simulink library "motor_interface_lib"  (R2022b)
settings: Solver=VariableStepAuto  StartTime=0.0  StopTime=10.0  RelTol=1e-3
undefined symbols (not defined in the file): MI_STATUSES
settings Model: Creator=dr_pa  LastModifiedBy=LinF

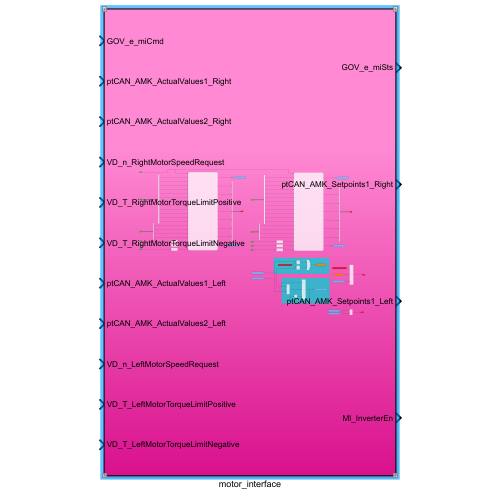
[thumbnail: Simulink's stored preview of the top-level diagram]
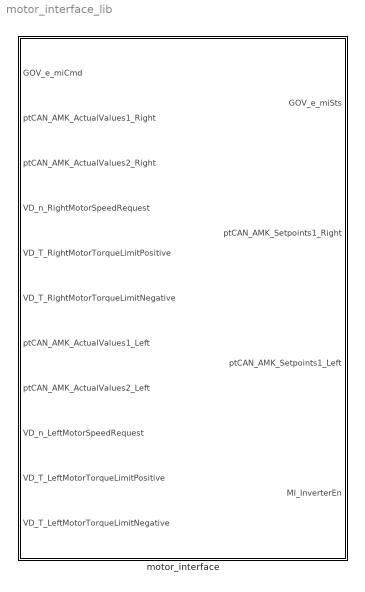
== system motor_interface_lib ==
  motor_interface : Subsystem

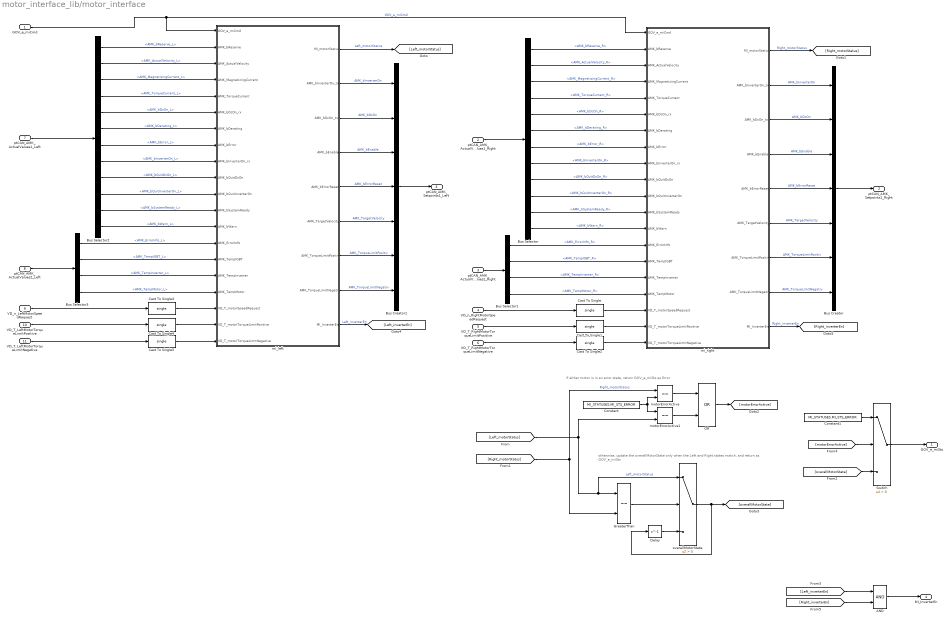
== system motor_interface_lib/motor_interface ==
  note: otherwise, update the overallMotorState only when the Left and Right states match, and return as GOV_e_miSts
  note: if either motor is in an error state, return GOV_e_miSts as Error
  GOV_e_miCmd : Inport
  ptCAN_AMK_ActualValues1_Right : Inport  Port=2
  ptCAN_AMK_ActualValues2_Right : Inport  Port=3
  VD_n_RightMotorSpeedRequest : Inport  Port=4
  VD_T_RightMotorTorqueLimitPositive : Inport  Port=5
  VD_T_RightMotorTorqueLimitNegative : Inport  Port=6
  ptCAN_AMK_ActualValues1_Left : Inport  Port=7
  ptCAN_AMK_ActualValues2_Left : Inport  Port=8
  VD_n_LeftMotorSpeedRequest : Inport  Port=9
  VD_T_LeftMotorTorqueLimitPositive : Inport  Port=10
  VD_T_LeftMotorTorqueLimitNegative : Inport  Port=11
  AND : Logic  AllPortsSameDT=off  OutDataTypeStr=boolean
  Bus Creator : BusCreator  Inputs=7
  Bus Creator1 : BusCreator  Inputs=7
  Bus Selector : BusSelector  OutputSignals=AMK_bReserve_R,AMK_ActualVelocity_R,AMK_MagnetizingCurrent_R,AMK_TorqueCurrent_R,AMK_bDcOn_R,AMK_bDerating_R,AMK_bError_R,AMK_bInverterOn_R,AMK_bQuitDcOn_R,AMK_bQuitInverterOn_R,AMK_bSystemReady_R,AMK_bWarn_R
  Bus Selector1 : BusSelector  OutputSignals=AMK_ErrorInfo_R,AMK_TempIGBT_R,AMK_TempInverter_R,AMK_TempMotor_R
  Bus Selector2 : BusSelector  OutputSignals=AMK_bReserve_L,AMK_ActualVelocity_L,AMK_MagnetizingCurrent_L,AMK_TorqueCurrent_L,AMK_bDcOn_L,AMK_bDerating_L,AMK_bError_L,AMK_bInverterOn_L,AMK_bQuitDcOn_L,AMK_bQuitInverterOn_L,AMK_bSystemReady_L,AMK_bWarn_L
  Bus Selector3 : BusSelector  OutputSignals=AMK_ErrorInfo_L,AMK_TempIGBT_L,AMK_TempInverter_L,AMK_TempMotor_L
  Cast To Single{,1..5} (6 alike) : DataTypeConversion  OutDataTypeStr=single  SaturateOnIntegerOverflow=off  RndMeth=Floor
  Constant : Constant  Value=MI_STATUSES.MI_STS_ERROR  OutDataTypeStr=Enum: MI_STATUSES
  Constant1 : Constant  Value=MI_STATUSES.MI_STS_ERROR  OutDataTypeStr=Enum: MI_STATUSES
  Delay : Delay  DelayLength=1  InitialCondition=MI_STATUSES.OFF
  GreaterThan : RelationalOperator  Operator===  OutDataTypeStr=boolean  RndMeth=Simplest  InputSameDT=off
  OR : Logic  Operator=OR  IconShape=distinctive  AllPortsSameDT=off  OutDataTypeStr=boolean
  Switch : Switch  Criteria=u2 > Threshold  SaturateOnIntegerOverflow=off  InputSameDT=off
  mi_left : Stateflow chart  TreatAsAtomicUnit=on
  mi_right : Stateflow chart  TreatAsAtomicUnit=on
  motorErrorActive : RelationalOperator  Operator===  OutDataTypeStr=boolean  RndMeth=Simplest  InputSameDT=off
  motorErrorActive1 : RelationalOperator  Operator===  OutDataTypeStr=boolean  RndMeth=Simplest  InputSameDT=off
  overallMotorState : Switch  Criteria=u2 > Threshold  SaturateOnIntegerOverflow=off  InputSameDT=off
  GOV_e_miSts : Outport
  ptCAN_AMK_Setpoints1_Right : Outport  Port=2
  ptCAN_AMK_Setpoints1_Left : Outport  Port=3
  MI_InverterEn : Outport  Port=4
  wires:
  [Right_inverterEn] -> AND/2
  [Left_inverterEn] -> AND/1
  mi_right/9(MI_InverterEn) -> [Right_inverterEn]  "Right_inverterEn"
  mi_left/9(MI_InverterEn) -> [Left_inverterEn]  "Left_inverterEn"
  AND/1 -> MI_InverterEn/1
  Bus Selector3/4 -> mi_left/17(AMK_TempMotor)  "<AMK_TempMotor_L>"
  Bus Selector3/3 -> mi_left/16(AMK_TempInverter)  "<AMK_TempInverter_L>"
  Bus Selector3/2 -> mi_left/15(AMK_TempIGBT)  "<AMK_TempIGBT_L>"
  Bus Selector3/1 -> mi_left/14(AMK_ErrorInfo)  "<AMK_ErrorInfo_L>"
  Bus Selector2/12 -> mi_left/13(AMK_bWarn)  "<AMK_bWarn_L>"
  Bus Selector2/11 -> mi_left/12(AMK_bSystemReady)  "<AMK_bSystemReady_L>"
  Bus Selector2/10 -> mi_left/11(AMK_bQuitInverterOn)  "<AMK_bQuitInverterOn_L>"
  Bus Selector2/9 -> mi_left/10(AMK_bQuitDcOn)  "<AMK_bQuitDcOn_L>"
  Bus Selector2/8 -> mi_left/9(AMK_bInverterOn_rx)  "<AMK_bInverterOn_L>"
  Bus Selector2/7 -> mi_left/8(AMK_bError)  "<AMK_bError_L>"
  Bus Selector2/6 -> mi_left/7(AMK_bDerating)  "<AMK_bDerating_L>"
  Bus Selector2/5 -> mi_left/6(AMK_bDcOn_rx)  "<AMK_bDcOn_L>"
  Bus Selector2/4 -> mi_left/5(AMK_TorqueCurrent)  "<AMK_TorqueCurrent_L>"
  Bus Selector2/3 -> mi_left/4(AMK_MagnetizingCurrent)  "<AMK_MagnetizingCurrent_L>"
  Bus Selector2/2 -> mi_left/3(AMK_ActualVelocity)  "<AMK_ActualVelocity_L>"
  Cast To Single5/1 -> mi_left/20(VD_T_motorTorqueLimitNegative)
  Cast To Single4/1 -> mi_left/19(VD_T_motorTorqueLimitPositive)
  Cast To Single3/1 -> mi_left/18(VD_T_motorSpeedRequest)
  Cast To Single2/1 -> mi_right/20(VD_T_motorTorqueLimitNegative)
  Cast To Single1/1 -> mi_right/19(VD_T_motorTorqueLimitPositive)
  Cast To Single/1 -> mi_right/18(VD_T_motorSpeedRequest)
  GOV_e_miCmd/1 -> mi_left/1(GOV_e_miCmd), mi_right/1(GOV_e_miCmd)  "GOV_e_miCmd"
  ptCAN_AMK_ActualValues1_Right/1 -> Bus Selector/1
  Bus Selector/2 -> mi_right/3(AMK_ActualVelocity)  "<AMK_ActualVelocity_R>"
  Bus Selector/3 -> mi_right/4(AMK_MagnetizingCurrent)  "<AMK_MagnetizingCurrent_R>"
  Bus Selector/4 -> mi_right/5(AMK_TorqueCurrent)  "<AMK_TorqueCurrent_R>"
  Bus Selector/5 -> mi_right/6(AMK_bDcOn_rx)  "<AMK_bDcOn_R>"
  Bus Selector/6 -> mi_right/7(AMK_bDerating)  "<AMK_bDerating_R>"
  Bus Selector/7 -> mi_right/8(AMK_bError)  "<AMK_bError_R>"
  Bus Selector/8 -> mi_right/9(AMK_bInverterOn_rx)  "<AMK_bInverterOn_R>"
  Bus Selector/9 -> mi_right/10(AMK_bQuitDcOn)  "<AMK_bQuitDcOn_R>"
  Bus Selector/10 -> mi_right/11(AMK_bQuitInverterOn)  "<AMK_bQuitInverterOn_R>"
  Bus Selector/11 -> mi_right/12(AMK_bSystemReady)  "<AMK_bSystemReady_R>"
  Bus Selector/12 -> mi_right/13(AMK_bWarn)  "<AMK_bWarn_R>"
  Bus Selector/1 -> mi_right/2(AMK_bReserve)  "<AMK_bReserve_R>"
  ptCAN_AMK_ActualValues2_Right/1 -> Bus Selector1/1
  Bus Selector1/1 -> mi_right/14(AMK_ErrorInfo)  "<AMK_ErrorInfo_R>"
  Bus Selector1/2 -> mi_right/15(AMK_TempIGBT)  "<AMK_TempIGBT_R>"
  Bus Selector1/3 -> mi_right/16(AMK_TempInverter)  "<AMK_TempInverter_R>"
  Bus Selector1/4 -> mi_right/17(AMK_TempMotor)  "<AMK_TempMotor_R>"
  Bus Creator/1 -> ptCAN_AMK_Setpoints1_Right/1
  mi_right/2(AMK_bInverterOn_tx) -> Bus Creator/1  "AMK_bInverterOn"
  mi_right/4(AMK_bEnable) -> Bus Creator/3  "AMK_bEnable"
  mi_right/6(AMK_TargetVelocity) -> Bus Creator/5  "AMK_TargetVelocity"
  mi_right/3(AMK_bDcOn_tx) -> Bus Creator/2  "AMK_bDcOn"
  mi_right/5(AMK_bErrorReset) -> Bus Creator/4  "AMK_bErrorReset"
  mi_left/1(MI_motorStatus) -> [Left_motorStatus]  "Left_motorStatus"
  mi_right/1(MI_motorStatus) -> [Right_motorStatus]  "Right_motorStatus"
  [Left_motorStatus] -> motorErrorActive1/2, overallMotorState/1, GreaterThan/1  "Left_motorStatus"
  [Right_motorStatus] -> motorErrorActive/1, GreaterThan/2  "Right_motorStatus"
  Constant/1 -> motorErrorActive/2, motorErrorActive1/1
  Switch/1 -> GOV_e_miSts/1
  [motorErrorActive] -> Switch/2
  overallMotorState/1 -> Delay/1, [overallMotorState]
  Delay/1 -> overallMotorState/3
  GreaterThan/1 -> overallMotorState/2
  [overallMotorState] -> Switch/3
  OR/1 -> [motorErrorActive]
  motorErrorActive1/1 -> OR/2
  motorErrorActive/1 -> OR/1
  Constant1/1 -> Switch/1
  mi_right/7(AMK_TorqueLimitPositiv) -> Bus Creator/6  "AMK_TorqueLimitPositiv"
  mi_right/8(AMK_TorqueLimitNegativ) -> Bus Creator/7  "AMK_TorqueLimitNegativ"
  VD_T_RightMotorTorqueLimitPositive/1 -> Cast To Single1/1
  VD_T_RightMotorTorqueLimitNegative/1 -> Cast To Single2/1
  VD_n_RightMotorSpeedRequest/1 -> Cast To Single/1
  VD_n_LeftMotorSpeedRequest/1 -> Cast To Single3/1
  VD_T_LeftMotorTorqueLimitNegative/1 -> Cast To Single5/1
  VD_T_LeftMotorTorqueLimitPositive/1 -> Cast To Single4/1
  Bus Selector2/1 -> mi_left/2(AMK_bReserve)  "<AMK_bReserve_L>"
  ptCAN_AMK_ActualValues1_Left/1 -> Bus Selector2/1
  mi_left/8(AMK_TorqueLimitNegativ) -> Bus Creator1/7  "AMK_TorqueLimitNegativ"
  mi_left/7(AMK_TorqueLimitPositiv) -> Bus Creator1/6  "AMK_TorqueLimitPositiv"
  mi_left/5(AMK_bErrorReset) -> Bus Creator1/4  "AMK_bErrorReset"
  mi_left/3(AMK_bDcOn_tx) -> Bus Creator1/2  "AMK_bDcOn"
  mi_left/6(AMK_TargetVelocity) -> Bus Creator1/5  "AMK_TargetVelocity"
  mi_left/4(AMK_bEnable) -> Bus Creator1/3  "AMK_bEnable"
  mi_left/2(AMK_bInverterOn_tx) -> Bus Creator1/1  "AMK_bInverterOn"
  Bus Creator1/1 -> ptCAN_AMK_Setpoints1_Left/1
  ptCAN_AMK_ActualValues2_Left/1 -> Bus Selector3/1

== stateflow chart motor_interface_lib/motor_interface/mi_left ==
  state motorOff_waitingForGov
    en:
    MI_motorStatus = MI_STATUSES.OFF;
    AMK_bInverterOn_tx = 0;
    AMK_bDcOn_tx = 0;
    AMK_bEnable = 0;
    AMK_bErrorReset = 0;
    AMK_TargetVelocity = 0;
    AMK_TorqueLimitPositiv = 0;
    AMK_TorqueLimitNegativ = 0;
    MI_InverterEn = 0;
  state AMK_startup
    state waiting_sysReady
      en:
      MI_motorStatus = MI_STATUSES.STARTUP;
    state toggleDCon
      en:
      AMK_bDcOn_tx = 1;
    state enforceSetpointsZero
      en:
      AMK_TargetVelocity = 0;
      AMK_TorqueLimitPositiv = 0;
      AMK_TorqueLimitNegativ = 0;
    state commandOn
      en:
      AMK_bEnable = 1;
      AMK_bInverterOn_tx = 1;
    waiting_sysReady -> (junction 67) [order 2] : [AMK_bError==1]
    waiting_sysReady -> toggleDCon [order 1] : [AMK_bSystemReady==1]
    toggleDCon -> (junction 67) [order 2] : [AMK_bError==1]
    toggleDCon -> AMK_startup.enforceSetpointsZero [order 1] : [(AMK_bDcOn_rx==1) ...
        | && (AMK_bQuitDcOn==1)]
    AMK_startup.enforceSetpointsZero -> (junction 67) [order 2] : [AMK_bError==1]
    commandOn -> (junction 67) [order 2] : [AMK_bError==1]
    AMK_startup.enforceSetpointsZero -> commandOn [order 1] : after(100,msec)
  state AMK_errorReset
    state toggleReset
      en:
      AMK_bErrorReset = 0;
    state sendReset
      en:
      AMK_bErrorReset = 1;
    state toggleEnable
      en:
      AMK_bEnable = 0;
    state enforceSetpointsZero
      en:
      AMK_TargetVelocity = 0;
      AMK_TorqueLimitPositiv = 0;
      AMK_TorqueLimitNegativ = 0;
      AMK_bInverterOn_tx = 0;
    sendReset -> toggleReset : after(500,msec)
    toggleEnable -> sendReset : after(500,msec)
    AMK_errorReset.enforceSetpointsZero -> toggleEnable : [AMK_bInverterOn_rx==0]
  state AMK_shutdown
    en:
    AMK_TargetVelocity = 0;
    AMK_TorqueLimitPositiv = 0;
    AMK_TorqueLimitNegativ = 0;
    MI_InverterEn = 0;
  state AMK_errorDetected
    en:
    MI_motorStatus = MI_STATUSES.MI_STS_ERROR;
  state AMK_ready
    en, du:
    MI_motorStatus = MI_STATUSES.READY;
    MI_InverterEn = 1;
  state AMK_running
    during:
    MI_motorStatus = MI_STATUSES.RUNNING;
    AMK_TargetVelocity = VD_T_motorSpeedRequest;
    AMK_TorqueLimitPositiv = VD_T_motorTorqueLimitPositive;
    AMK_TorqueLimitNegativ = VD_T_motorTorqueLimitNegative;
  toggleReset -> motorOff_waitingForGov : [AMK_bSystemReady==1]
  commandOn -> AMK_ready [order 1] : [AMK_bInverterOn_rx ==1]
  motorOff_waitingForGov -> waiting_sysReady : [GOV_e_miCmd == MI_CMD.CMD_STARTUP]
  (default) -> motorOff_waitingForGov
  (junction 67) -> AMK_errorDetected
  AMK_shutdown -> motorOff_waitingForGov : after(500,msec)
  AMK_running -> AMK_shutdown [order 2] : [GOV_e_miCmd == MI_CMD.CMD_SHUTDOWN]
  AMK_errorDetected -> AMK_errorReset.enforceSetpointsZero : [GOV_e_miCmd == MI_CMD.ERR_RESET]
  AMK_ready -> AMK_errorDetected [order 1] : [AMK_bError==1]
  AMK_running -> AMK_errorDetected [order 1] : [AMK_bError==1]
  AMK_ready -> AMK_running [order 2] : [(AMK_bQuitInverterOn == 1) && ...
      | (AMK_bError == 0)]
  data: GOV_e_miCmd input Enum: MI_CMD; AMK_bReserve input; AMK_ActualVelocity input; AMK_MagnetizingCurrent input; AMK_TorqueCurrent input; AMK_bDcOn_rx input; AMK_bDerating input; AMK_bError input; AMK_bInverterOn_rx input; AMK_bQuitDcOn input; AMK_bQuitInverterOn input; MI_motorStatus output Enum: MI_STATUSES size=1; AMK_bSystemReady input; AMK_bWarn input; AMK_ErrorInfo input; AMK_TempIGBT input; AMK_TempInverter input; AMK_TempMotor input; VD_T_motorSpeedRequest input; AMK_bInverterOn_tx output uint8 size=1; AMK_bDcOn_tx output uint8 size=1; AMK_bEnable output uint8 size=1; AMK_bErrorReset output uint8 size=1; AMK_TargetVelocity output single size=1; AMK_TorqueLimitPositiv output single size=1; AMK_TorqueLimitNegativ output single size=1; VD_T_motorTorqueLimitPositive input; VD_T_motorTorqueLimitNegative input; MI_InverterEn output

== stateflow chart motor_interface_lib/motor_interface/mi_right ==
  state motorOff_waitingForGov
    en:
    MI_motorStatus = MI_STATUSES.OFF;
    AMK_bInverterOn_tx = 0;
    AMK_bDcOn_tx = 0;
    AMK_bEnable = 0;
    AMK_bErrorReset = 0;
    AMK_TargetVelocity = 0;
    AMK_TorqueLimitPositiv = 0;
    AMK_TorqueLimitNegativ = 0;
    MI_InverterEn = 0;
  state AMK_startup
    state waiting_sysReady
      en:
      MI_motorStatus = MI_STATUSES.STARTUP;
    state toggleDCon
      en:
      AMK_bDcOn_tx = 1;
    state enforceSetpointsZero
      en:
      AMK_TargetVelocity = 0;
      AMK_TorqueLimitPositiv = 0;
      AMK_TorqueLimitNegativ = 0;
    state commandOn
      en:
      AMK_bEnable = 1;
      AMK_bInverterOn_tx = 1;
    waiting_sysReady -> (junction 67) [order 2] : [AMK_bError==1]
    waiting_sysReady -> toggleDCon [order 1] : [AMK_bSystemReady==1]
    toggleDCon -> (junction 67) [order 2] : [AMK_bError==1]
    toggleDCon -> AMK_startup.enforceSetpointsZero [order 1] : [(AMK_bDcOn_rx==1) ...
        | && (AMK_bQuitDcOn==1)]
    AMK_startup.enforceSetpointsZero -> (junction 67) [order 2] : [AMK_bError==1]
    commandOn -> (junction 67) [order 2] : [AMK_bError==1]
    AMK_startup.enforceSetpointsZero -> commandOn [order 1] : after(100,msec)
  state AMK_errorReset
    state toggleReset
      en:
      AMK_bErrorReset = 0;
    state sendReset
      en:
      AMK_bErrorReset = 1;
    state toggleEnable
      en:
      AMK_bEnable = 0;
    state enforceSetpointsZero
      en:
      AMK_TargetVelocity = 0;
      AMK_TorqueLimitPositiv = 0;
      AMK_TorqueLimitNegativ = 0;
      AMK_bInverterOn_tx = 0;
    sendReset -> toggleReset : after(500,msec)
    toggleEnable -> sendReset : after(500,msec)
    AMK_errorReset.enforceSetpointsZero -> toggleEnable : [AMK_bInverterOn_rx==0]
  state AMK_shutdown
    en:
    AMK_TargetVelocity = 0;
    AMK_TorqueLimitPositiv = 0;
    AMK_TorqueLimitNegativ = 0;
    MI_InverterEn = 0;
  state AMK_errorDetected
    en:
    MI_motorStatus = MI_STATUSES.MI_STS_ERROR;
  state AMK_ready
    en, du:
    MI_motorStatus = MI_STATUSES.READY;
    MI_InverterEn = 1;
  state AMK_running
    during:
    MI_motorStatus = MI_STATUSES.RUNNING;
    AMK_TargetVelocity = VD_T_motorSpeedRequest;
    AMK_TorqueLimitPositiv = VD_T_motorTorqueLimitPositive;
    AMK_TorqueLimitNegativ = VD_T_motorTorqueLimitNegative;
  toggleReset -> motorOff_waitingForGov : [AMK_bSystemReady==1]
  commandOn -> AMK_ready [order 1] : [AMK_bInverterOn_rx ==1]
  motorOff_waitingForGov -> waiting_sysReady : [GOV_e_miCmd == MI_CMD.CMD_STARTUP]
  (default) -> motorOff_waitingForGov
  (junction 67) -> AMK_errorDetected
  AMK_shutdown -> motorOff_waitingForGov : after(500,msec)
  AMK_running -> AMK_shutdown [order 2] : [GOV_e_miCmd == MI_CMD.CMD_SHUTDOWN]
  AMK_errorDetected -> AMK_errorReset.enforceSetpointsZero : [GOV_e_miCmd == MI_CMD.ERR_RESET]
  AMK_ready -> AMK_errorDetected [order 1] : [AMK_bError==1]
  AMK_running -> AMK_errorDetected [order 1] : [AMK_bError==1]
  AMK_ready -> AMK_running [order 2] : [(AMK_bQuitInverterOn == 1) && ...
      | (AMK_bError == 0)]
  data: GOV_e_miCmd input Enum: MI_CMD; AMK_bReserve input; AMK_ActualVelocity input; AMK_MagnetizingCurrent input; AMK_TorqueCurrent input; AMK_bDcOn_rx input; AMK_bDerating input; AMK_bError input; AMK_bInverterOn_rx input; AMK_bQuitDcOn input; AMK_bQuitInverterOn input; MI_motorStatus output Enum: MI_STATUSES size=1; AMK_bSystemReady input; AMK_bWarn input; AMK_ErrorInfo input; AMK_TempIGBT input; AMK_TempInverter input; AMK_TempMotor input; VD_T_motorSpeedRequest input; AMK_bInverterOn_tx output uint8 size=1; AMK_bDcOn_tx output uint8 size=1; AMK_bEnable output uint8 size=1; AMK_bErrorReset output uint8 size=1; AMK_TargetVelocity output single size=1; AMK_TorqueLimitPositiv output single size=1; AMK_TorqueLimitNegativ output single size=1; VD_T_motorTorqueLimitPositive input; VD_T_motorTorqueLimitNegative input; MI_InverterEn output
